simulink model "LotkaVolterra"  (R2016a)
settings: Solver=VariableStepAuto  StartTime=0.0  StopTime=10.0  RelTol=1e-6
settings Model: Creator=paulotabuada  LastModifiedBy=paulotabuada

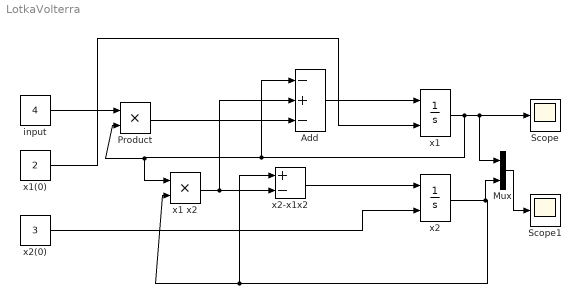
== system LotkaVolterra ==
  Add : Sum  Inputs=-+-
  Mux : Mux  Inputs=2
  Product : Product
  Scope : Scope
  Scope1 : Scope
  input : Constant  Value=4
  x1 : Integrator  InitialConditionSource=external
  x1 x2 : Product
  x1(0) : Constant  Value=2
  x2 : Integrator  InitialConditionSource=external
  x2(0) : Constant  Value=3
  x2-x1x2 : Sum  Inputs=+-
  wires:
  x2-x1x2/1 -> x2/1
  x2/1 -> Mux/2, x1 x2/2, x2-x1x2/1
  x1 x2/1 -> Add/2, x2-x1x2/2
  x1/1 -> Mux/1, Scope/1, Add/1, Product/2, x1 x2/1
  Add/1 -> x1/1
  Product/1 -> Add/3
  input/1 -> Product/1
  x1(0)/1 -> x1/2
  x2(0)/1 -> x2/2
  Mux/1 -> Scope1/1
